simulink model "RefModel_Task"  (R2015b)
settings: configuration reference "CenterOutReachConfigSet" (kept outside this file)
undefined symbols (not defined in the file or in its folder): SimulinkParameter_TunableConditionRepeats, SimulinkParameter_TunableConditions, SimulinkParameter_TunableDataLoggerInfo, SimulinkParameter_TunableNextTrialId, SimulinkParameter_TunableParam, SimulinkParameter_TunableTaskControl
libraries: libBusSerialize x7, libUtilities x1, dspsrcs4 x1
(part 3 of 3)

== matlab function RefModel_Task/Tunable Task Control/Deserialize Bus Parameter ==
  data: valAsDouble input double; bus output Bus: TaskControlBus size=1; update output uint8 size=1; allowPending input uint8 size=1; receivedInvalid output uint8 size=1
function [bus, update, receivedInvalid] = deserializeBusParameter(valAsDouble, allowPending)
%#codegen

    % typecast to bytes
    valAsBytes = typecast(valAsDouble, 'uint8');

    % use the first byte as updateCounter, check for whether counter has been incremented
    thisCounter = valAsBytes(1);
    persistent pLastCounter;
    if isempty(pLastCounter)
        pLastCounter = thisCounter;
    end
    if pLastCounter ~= thisCounter
        recvUpdate = uint8(1);
        pLastCounter = thisCounter;
    else
        recvUpdate = uint8(0);
    end
    startOffset = 2;

    % external cached output for when allowPending 
    persistent pBusOut;
    if isempty(pBusOut)
        pBusOut = initializeBus_TaskControlBus();
    end

    % parse incoming bytes if allowing updates
    receivedInvalid = uint8(0);
    if allowPending
        [bus, valid] = deserializeBus_TaskControlBus(valAsBytes, startOffset);
        if valid
            % update internal cache
            pBusOut = bus;
        else
            % don't update internal cache, output internal cache
            bus = pBusOut;
            receivedInvalid = uint8(1);
            recvUpdate = uint8(0);
        end
    else
        bus = pBusOut;
    end

    % track whether we have a pending update
    persistent pPending;
    if isempty(pPending), pPending = uint8(0); end
    if recvUpdate
        if allowPending
            % update goes out immediately
            update = uint8(1);
            pPending = uint8(0);
        else
            % queue pending update
            update = uint8(0);
            pPending = uint8(1);
        end
    else
        if allowPending
            % release pending
            update = pPending;
            pPending = uint8(0);
        else
            % do nothing
            update = uint8(0);
        end
    end

    % reset fields marked with .resetImmediately immediately after update
    if ~update
        bus.endTimeoutNow = uint8(0);
        bus.giveFreeJuice = uint8(0);
        bus.resetConditionBlock = uint8(0);

    end
end

== matlab function RefModel_Task/Tunable Serialized Conditions Array/Deserialize Parameter ==
  data: valAsDouble input double; value output uint8 size=16562; update output uint8 size=1
function [value, update] = deserializeParameter(valAsDouble)
%#codegen

valAsBytes = typecast(valAsDouble, 'uint8');

% check for whether counter has been incremented
thisCounter = valAsBytes(1);
persistent pLastCounter;
if isempty(pLastCounter)
    pLastCounter = thisCounter;
end
if pLastCounter ~= thisCounter
    update = uint8(1);
    pLastCounter = thisCounter;
else
    update = uint8(0);
end

% typecast and reshape the value
value = reshape(typecast(valAsBytes(double(2):double(16563)), 'uint8'), [16562 1]);
